simulink model "SPWM_HDLCoder_MCSI2024"  (R2021a)
settings: Solver=FixedStepDiscrete  StartTime=0.0  StopTime=0.00001  FixedStep=2.5e-8  RelTol=1e-3  EnableMultiTasking=on
undefined symbols (not defined in the file or in its folder): cfg
libraries: simulink x9, hdlsllib x8
settings Model: Creator=Damian  LastModifiedBy=Damian
settings OptimizationCC: BlockReduction=off  ConditionallyExecuteInputs=off
settings DebuggingCC: SingleTaskRateTransMsg=error

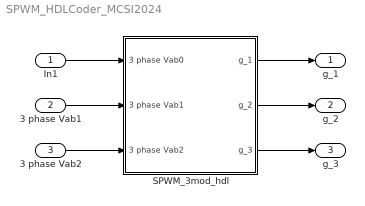
== system SPWM_HDLCoder_MCSI2024 ==
  In1 : Inport  OutDataTypeStr=fixdt(0,8,0)
  3 phase Vab1 : Inport  Port=2  OutDataTypeStr=fixdt(0,8,0)
  3 phase Vab2 : Inport  Port=3  OutDataTypeStr=fixdt(0,8,0)
  SPWM_3mod_hdl : Subsystem
  g_1 : Outport
  g_2 : Outport  Port=2
  g_3 : Outport  Port=3
  wires:
  In1/1 -> SPWM_3mod_hdl/1(3 phase Vab0)
  3 phase Vab1/1 -> SPWM_3mod_hdl/2(3 phase Vab1)
  3 phase Vab2/1 -> SPWM_3mod_hdl/3(3 phase Vab2)
  SPWM_3mod_hdl/1(g_1) -> g_1/1
  SPWM_3mod_hdl/2(g_2) -> g_2/1
  SPWM_3mod_hdl/3(g_3) -> g_3/1

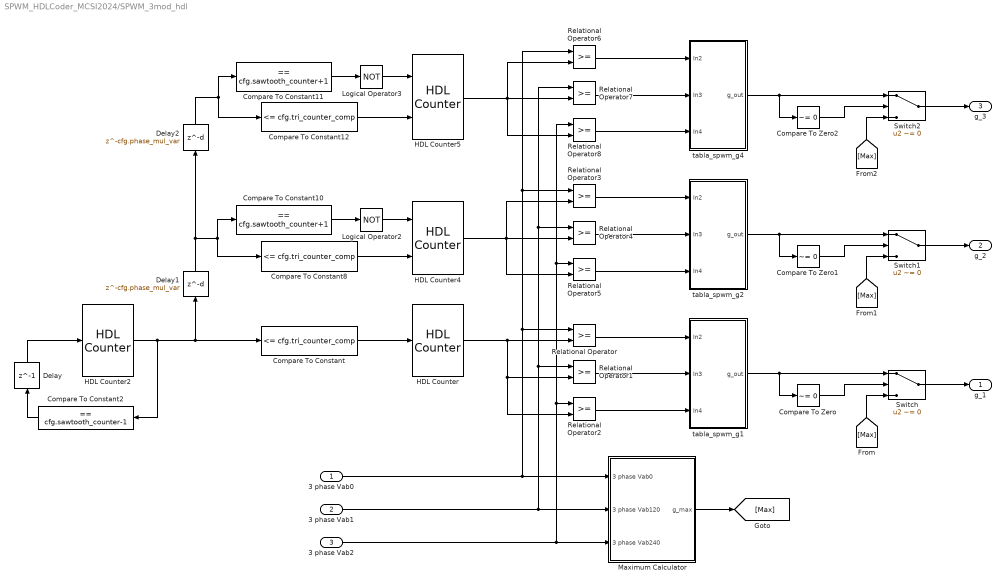
== system SPWM_HDLCoder_MCSI2024/SPWM_3mod_hdl ==
  3 phase Vab0 : Inport  OutDataTypeStr=fixdt(0,8,0)
  3 phase Vab1 : Inport  Port=2  OutDataTypeStr=fixdt(0,8,0)
  3 phase Vab2 : Inport  Port=3  OutDataTypeStr=fixdt(0,8,0)
  Compare To Constant : simulink/Logic and Bit Operations/Compare To Constant  relop=<=  const=cfg.tri_counter_comp  OutDataTypeStr=boolean
  Compare To Constant10 : simulink/Logic and Bit Operations/Compare To Constant  relop===  const=cfg.sawtooth_counter+1  OutDataTypeStr=boolean
  Compare To Constant11 : simulink/Logic and Bit Operations/Compare To Constant  relop===  const=cfg.sawtooth_counter+1  OutDataTypeStr=boolean
  Compare To Constant12 : simulink/Logic and Bit Operations/Compare To Constant  relop=<=  const=cfg.tri_counter_comp  OutDataTypeStr=boolean
  Compare To Constant2 : simulink/Logic and Bit Operations/Compare To Constant  relop===  const=cfg.sawtooth_counter-1  OutDataTypeStr=boolean
  Compare To Constant8 : simulink/Logic and Bit Operations/Compare To Constant  relop=<=  const=cfg.tri_counter_comp  OutDataTypeStr=boolean
  Compare To Zero : simulink/Logic and Bit Operations/Compare To Zero  relop=~=  OutDataTypeStr=boolean
  Compare To Zero1 : simulink/Logic and Bit Operations/Compare To Zero  relop=~=  OutDataTypeStr=boolean
  Compare To Zero2 : simulink/Logic and Bit Operations/Compare To Zero  relop=~=  OutDataTypeStr=boolean
  Delay : Delay  DelayLength=1  InitialCondition=0
  Delay1 : Delay  DelayLength=cfg.phase_mul_var  InitialCondition=cfg.sawtooth_counter+1
  Delay2 : Delay  DelayLength=cfg.phase_mul_var  InitialCondition=cfg.sawtooth_counter+1
  HDL Counter : hdlsllib/Sources/HDL Counter  CountType=Free running  CountInit=0  CountStep=1  CountMax=255  CountFromType=Initial value  CountFrom=0  CountResetPort=off  CountLoadPort=off  CountEnbPort=off  CountDirPort=on  CountHitOutputPort=off  CountDataType=Unsigned  CountWordLen=8  CountFracLen=0  CountSampTime=1
  HDL Counter2 : hdlsllib/Sources/HDL Counter  CountType=Free running  CountInit=0  CountStep=1  CountMax=cfg.sawtooth_counter-1  CountFromType=Initial value  CountFrom=0  CountResetPort=on  CountLoadPort=off  CountEnbPort=off  CountDirPort=off  CountHitOutputPort=off  CountDataType=Unsigned  CountWordLen=16  CountFracLen=0  CountSampTime=1
  HDL Counter4 : hdlsllib/Sources/HDL Counter  CountType=Free running  CountInit=0  CountStep=1  CountMax=255  CountFromType=Initial value  CountFrom=0  CountResetPort=off  CountLoadPort=off  CountEnbPort=on  CountDirPort=on  CountHitOutputPort=off  CountDataType=Unsigned  CountWordLen=8  CountFracLen=0  CountSampTime=1
  HDL Counter5 : hdlsllib/Sources/HDL Counter  CountType=Free running  CountInit=0  CountStep=1  CountMax=255  CountFromType=Initial value  CountFrom=0  CountResetPort=off  CountLoadPort=off  CountEnbPort=on  CountDirPort=on  CountHitOutputPort=off  CountDataType=Unsigned  CountWordLen=8  CountFracLen=0  CountSampTime=1
  Logical Operator2 : Logic  Operator=NOT  AllPortsSameDT=off  OutDataTypeStr=boolean
  Logical Operator3 : Logic  Operator=NOT  AllPortsSameDT=off  OutDataTypeStr=boolean
  Maximum Calculator : Subsystem
  Relational Operator{,1..8} (9 alike) : RelationalOperator  OutDataTypeStr=boolean  RndMeth=Nearest
  Switch : Switch  Criteria=u2 ~= 0
  Switch1 : Switch  Criteria=u2 ~= 0
  Switch2 : Switch  Criteria=u2 ~= 0
  tabla_spwm_g1 : Subsystem
  tabla_spwm_g2 : Subsystem
  tabla_spwm_g4 : Subsystem
  g_1 : Outport
  g_2 : Outport  Port=2
  g_3 : Outport  Port=3
  wires:
  HDL Counter4/1 -> Relational Operator4/2, Relational Operator3/2, Relational Operator5/2
  Compare To Constant12/1 -> HDL Counter5/2
  tabla_spwm_g4/1(g_out) -> Compare To Zero2/1, Switch2/1
  3 phase Vab2/1 -> Relational Operator5/1, Relational Operator8/1, Relational Operator2/1, Maximum Calculator/3(3 phase Vab240)
  Delay1/1 -> Delay2/1, Compare To Constant10/1, Compare To Constant8/1
  [Max] -> Switch/3
  Relational Operator1/1 -> tabla_spwm_g1/2(In3)
  Delay2/1 -> Compare To Constant11/1, Compare To Constant12/1
  tabla_spwm_g1/1(g_out) -> Compare To Zero/1, Switch/1
  Relational Operator/1 -> tabla_spwm_g1/1(In2)
  Relational Operator7/1 -> tabla_spwm_g4/2(In3)
  Logical Operator2/1 -> HDL Counter4/1
  Relational Operator8/1 -> tabla_spwm_g4/3(In4)
  Delay/1 -> HDL Counter2/1
  3 phase Vab1/1 -> Maximum Calculator/2(3 phase Vab120), Relational Operator1/1, Relational Operator4/1, Relational Operator7/1
  Compare To Zero2/1 -> Switch2/2
  3 phase Vab0/1 -> Maximum Calculator/1(3 phase Vab0), Relational Operator/1, Relational Operator3/1, Relational Operator6/1
  Compare To Constant2/1 -> Delay/1
  [Max] -> Switch2/3
  Switch2/1 -> g_3/1
  Maximum Calculator/1(g_max) -> [Max]
  Relational Operator6/1 -> tabla_spwm_g4/1(In2)
  HDL Counter2/1 -> Compare To Constant2/1, Delay1/1, Compare To Constant/1
  HDL Counter5/1 -> Relational Operator7/2, Relational Operator6/2, Relational Operator8/2
  HDL Counter/1 -> Relational Operator2/2, Relational Operator1/2, Relational Operator/2
  Switch/1 -> g_1/1
  Compare To Constant10/1 -> Logical Operator2/1
  Compare To Zero/1 -> Switch/2
  Relational Operator5/1 -> tabla_spwm_g2/3(In4)
  Relational Operator2/1 -> tabla_spwm_g1/3(In4)
  Compare To Constant/1 -> HDL Counter/1
  tabla_spwm_g2/1(g_out) -> Compare To Zero1/1, Switch1/1
  [Max] -> Switch1/3
  Compare To Constant8/1 -> HDL Counter4/2
  Compare To Constant11/1 -> Logical Operator3/1
  Compare To Zero1/1 -> Switch1/2
  Logical Operator3/1 -> HDL Counter5/1
  Switch1/1 -> g_2/1
  Relational Operator3/1 -> tabla_spwm_g2/1(In2)
  Relational Operator4/1 -> tabla_spwm_g2/2(In3)

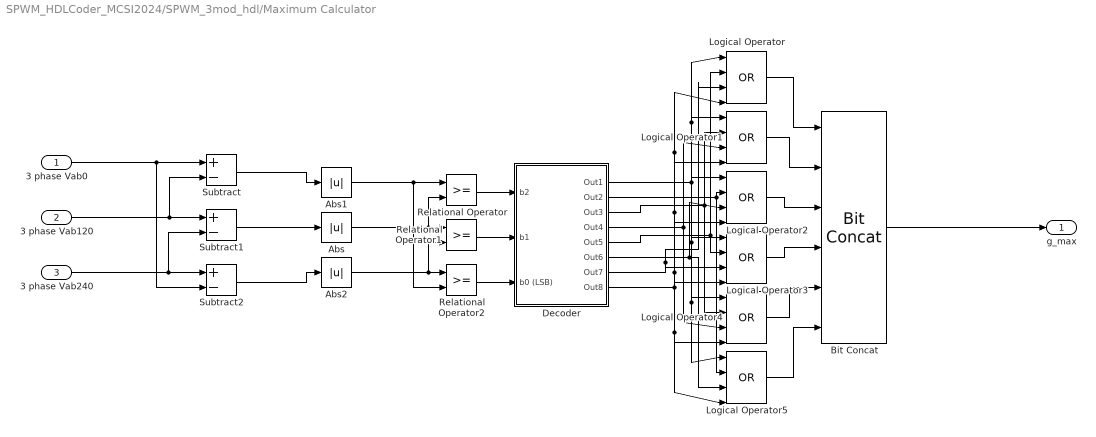
== system SPWM_HDLCoder_MCSI2024/SPWM_3mod_hdl/Maximum Calculator ==
  3 phase Vab0 : Inport
  3 phase Vab120 : Inport  Port=2
  3 phase Vab240 : Inport  Port=3
  Abs : Abs
  Abs1 : Abs
  Abs2 : Abs
  Bit Concat : hdlsllib/Logic and Bit Operations/Bit Concat  numInputs=6
  Decoder : Subsystem
  Logical Operator{,1..5} (6 alike) : Logic  Operator=OR  Inputs=4  IconShape=distinctive  AllPortsSameDT=off  OutDataTypeStr=boolean
  Relational Operator : RelationalOperator  OutDataTypeStr=boolean  RndMeth=Nearest
  Relational Operator1 : RelationalOperator  OutDataTypeStr=boolean  RndMeth=Nearest
  Relational Operator2 : RelationalOperator  OutDataTypeStr=boolean  RndMeth=Nearest
  Subtract : Sum  Inputs=+-  OutDataTypeStr=int16
  Subtract1 : Sum  Inputs=+-  OutDataTypeStr=int16
  Subtract2 : Sum  Inputs=+-  OutDataTypeStr=int16
  g_max : Outport  VectorParamsAs1DForOutWhenUnconnected=off
  wires:
  Relational Operator/1 -> Decoder/1(b2)
  Abs1/1 -> Relational Operator/1, Relational Operator2/2
  Logical Operator2/1 -> Bit Concat/3
  Abs/1 -> Relational Operator/2, Relational Operator1/1
  3 phase Vab0/1 -> Subtract2/2, Subtract/1
  Decoder/6(Out6) -> Logical Operator5/3, Logical Operator2/3
  Decoder/3(Out3) -> Logical Operator4/2, Logical Operator1/2
  Decoder/2(Out2) -> Logical Operator2/2, Logical Operator5/2
  3 phase Vab240/1 -> Subtract2/1, Subtract1/2
  Logical Operator5/1 -> Bit Concat/6
  Decoder/1(Out1) -> Logical Operator1/1, Logical Operator/1, Logical Operator5/1, Logical Operator4/1, Logical Operator3/1, Logical Operator2/1
  Abs2/1 -> Relational Operator1/2, Relational Operator2/1
  Subtract1/1 -> Abs/1
  Decoder/4(Out4) -> Logical Operator4/3, Logical Operator1/3
  3 phase Vab120/1 -> Subtract1/1, Subtract/2
  Logical Operator3/1 -> Bit Concat/4
  Decoder/5(Out5) -> Logical Operator3/2, Logical Operator/2
  Subtract/1 -> Abs1/1
  Subtract2/1 -> Abs2/1
  Relational Operator1/1 -> Decoder/2(b1)
  Relational Operator2/1 -> Decoder/3(b0 (LSB))
  Logical Operator1/1 -> Bit Concat/2
  Decoder/8(Out8) -> Logical Operator/4, Logical Operator1/4, Logical Operator2/4, Logical Operator3/4, Logical Operator4/4, Logical Operator5/4
  Decoder/7(Out7) -> Logical Operator3/3, Logical Operator/3
  Logical Operator4/1 -> Bit Concat/5
  Logical Operator/1 -> Bit Concat/1
  Bit Concat/1 -> g_max/1

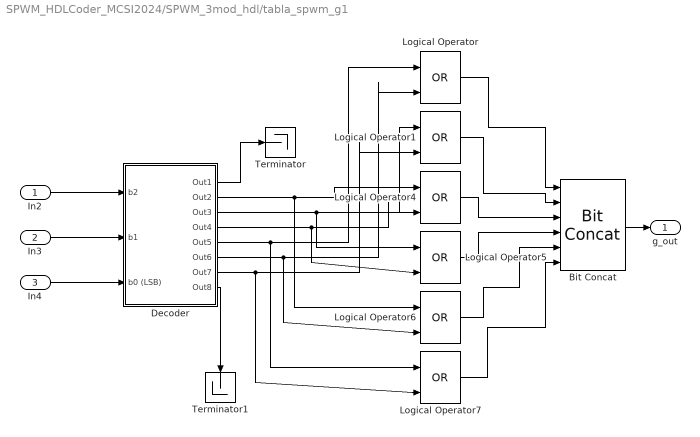
== system SPWM_HDLCoder_MCSI2024/SPWM_3mod_hdl/tabla_spwm_g1 ==
  In2 : Inport
  In3 : Inport  Port=2
  In4 : Inport  Port=3
  Bit Concat : hdlsllib/Logic and Bit Operations/Bit Concat  numInputs=6
  Decoder : Subsystem
  Logical Operator{,1,4..7} (6 alike) : Logic  Operator=OR  IconShape=distinctive  AllPortsSameDT=off  OutDataTypeStr=boolean
  Terminator : Terminator
  Terminator1 : Terminator
  g_out : Outport  VectorParamsAs1DForOutWhenUnconnected=off
  wires:
  Decoder/7(Out7) -> Logical Operator1/2, Logical Operator7/2
  Logical Operator4/1 -> Bit Concat/3
  Logical Operator/1 -> Bit Concat/1
  Logical Operator1/1 -> Bit Concat/2
  Decoder/2(Out2) -> Logical Operator4/1, Logical Operator6/1
  Logical Operator7/1 -> Bit Concat/6
  Logical Operator5/1 -> Bit Concat/4
  Decoder/5(Out5) -> Logical Operator/1, Logical Operator7/1
  Logical Operator6/1 -> Bit Concat/5
  In4/1 -> Decoder/3(b0 (LSB))
  In3/1 -> Decoder/2(b1)
  In2/1 -> Decoder/1(b2)
  Decoder/4(Out4) -> Logical Operator5/2, Logical Operator4/2
  Decoder/3(Out3) -> Logical Operator5/1, Logical Operator1/1
  Decoder/6(Out6) -> Logical Operator/2, Logical Operator6/2
  Decoder/1(Out1) -> Terminator/1
  Decoder/8(Out8) -> Terminator1/1
  Bit Concat/1 -> g_out/1

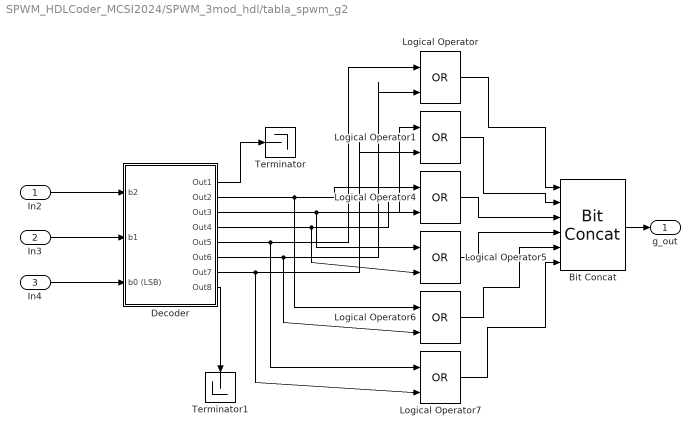
== system SPWM_HDLCoder_MCSI2024/SPWM_3mod_hdl/tabla_spwm_g2 ==
  In2 : Inport
  In3 : Inport  Port=2
  In4 : Inport  Port=3
  Bit Concat : hdlsllib/Logic and Bit Operations/Bit Concat  numInputs=6
  Decoder : Subsystem
  Logical Operator{,1,4..7} (6 alike) : Logic  Operator=OR  IconShape=distinctive  AllPortsSameDT=off  OutDataTypeStr=boolean
  Terminator : Terminator
  Terminator1 : Terminator
  g_out : Outport  VectorParamsAs1DForOutWhenUnconnected=off
  wires:
  Decoder/7(Out7) -> Logical Operator1/2, Logical Operator7/2
  Logical Operator4/1 -> Bit Concat/3
  Logical Operator/1 -> Bit Concat/1
  Logical Operator1/1 -> Bit Concat/2
  Decoder/2(Out2) -> Logical Operator4/1, Logical Operator6/1
  Logical Operator7/1 -> Bit Concat/6
  Logical Operator5/1 -> Bit Concat/4
  Decoder/5(Out5) -> Logical Operator/1, Logical Operator7/1
  Logical Operator6/1 -> Bit Concat/5
  In4/1 -> Decoder/3(b0 (LSB))
  In3/1 -> Decoder/2(b1)
  In2/1 -> Decoder/1(b2)
  Decoder/4(Out4) -> Logical Operator5/2, Logical Operator4/2
  Decoder/3(Out3) -> Logical Operator5/1, Logical Operator1/1
  Decoder/6(Out6) -> Logical Operator/2, Logical Operator6/2
  Decoder/1(Out1) -> Terminator/1
  Decoder/8(Out8) -> Terminator1/1
  Bit Concat/1 -> g_out/1

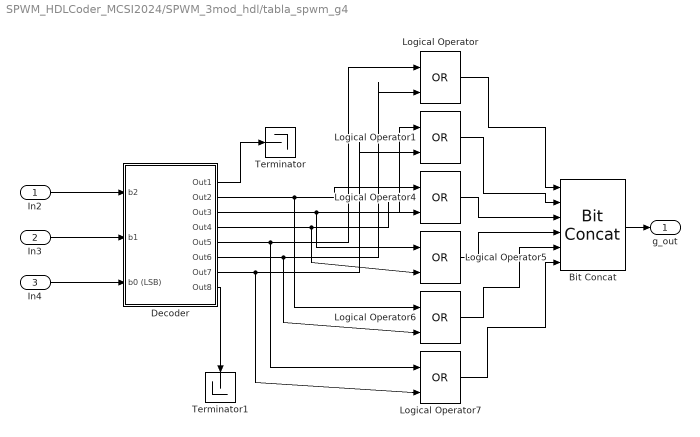
== system SPWM_HDLCoder_MCSI2024/SPWM_3mod_hdl/tabla_spwm_g4 ==
  In2 : Inport
  In3 : Inport  Port=2
  In4 : Inport  Port=3
  Bit Concat : hdlsllib/Logic and Bit Operations/Bit Concat  numInputs=6
  Decoder : Subsystem
  Logical Operator{,1,4..7} (6 alike) : Logic  Operator=OR  IconShape=distinctive  AllPortsSameDT=off  OutDataTypeStr=boolean
  Terminator : Terminator
  Terminator1 : Terminator
  g_out : Outport  VectorParamsAs1DForOutWhenUnconnected=off
  wires:
  Decoder/7(Out7) -> Logical Operator1/2, Logical Operator7/2
  Logical Operator4/1 -> Bit Concat/3
  Logical Operator/1 -> Bit Concat/1
  Logical Operator1/1 -> Bit Concat/2
  Decoder/2(Out2) -> Logical Operator4/1, Logical Operator6/1
  Logical Operator7/1 -> Bit Concat/6
  Logical Operator5/1 -> Bit Concat/4
  Decoder/5(Out5) -> Logical Operator/1, Logical Operator7/1
  Logical Operator6/1 -> Bit Concat/5
  In4/1 -> Decoder/3(b0 (LSB))
  In3/1 -> Decoder/2(b1)
  In2/1 -> Decoder/1(b2)
  Decoder/4(Out4) -> Logical Operator5/2, Logical Operator4/2
  Decoder/3(Out3) -> Logical Operator5/1, Logical Operator1/1
  Decoder/6(Out6) -> Logical Operator/2, Logical Operator6/2
  Decoder/1(Out1) -> Terminator/1
  Decoder/8(Out8) -> Terminator1/1
  Bit Concat/1 -> g_out/1

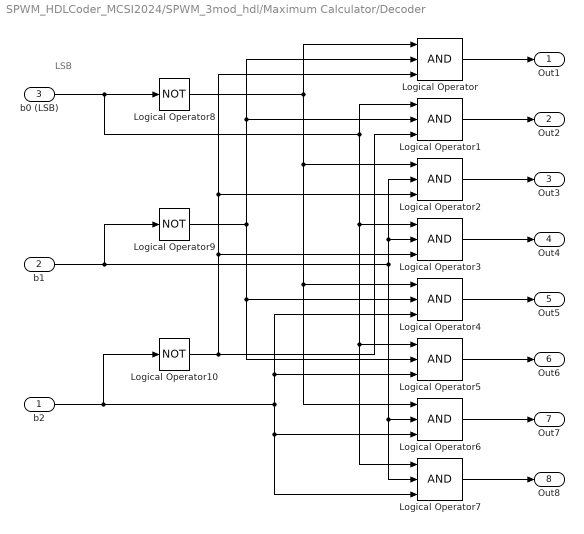
== system SPWM_HDLCoder_MCSI2024/SPWM_3mod_hdl/Maximum Calculator/Decoder ==
  note: LSB
  b2 : Inport
  b1 : Inport  Port=2
  b0 (LSB) : Inport  Port=3
  Logical Operator{,1..7} (8 alike) : Logic  Inputs=3  IconShape=distinctive  AllPortsSameDT=off  OutDataTypeStr=boolean
  Logical Operator10 : Logic  Operator=NOT  IconShape=distinctive  AllPortsSameDT=off  OutDataTypeStr=boolean
  Logical Operator8 : Logic  Operator=NOT  IconShape=distinctive  AllPortsSameDT=off  OutDataTypeStr=boolean
  Logical Operator9 : Logic  Operator=NOT  IconShape=distinctive  AllPortsSameDT=off  OutDataTypeStr=boolean
  Out1 : Outport
  Out2 : Outport  Port=2
  Out3 : Outport  Port=3
  Out4 : Outport  Port=4
  Out5 : Outport  Port=5
  Out6 : Outport  Port=6
  Out7 : Outport  Port=7
  Out8 : Outport  Port=8
  wires:
  Logical Operator9/1 -> Logical Operator5/2, Logical Operator4/2, Logical Operator1/2, Logical Operator/2
  Logical Operator5/1 -> Out6/1
  Logical Operator1/1 -> Out2/1
  Logical Operator10/1 -> Logical Operator3/3, Logical Operator2/3, Logical Operator/3, Logical Operator1/3
  Logical Operator/1 -> Out1/1
  Logical Operator8/1 -> Logical Operator6/1, Logical Operator4/1, Logical Operator2/1, Logical Operator/1
  b2/1 -> Logical Operator4/3, Logical Operator5/3, Logical Operator7/3, Logical Operator6/3, Logical Operator10/1
  b0 (LSB)/1 -> Logical Operator7/1, Logical Operator5/1, Logical Operator3/1, Logical Operator1/1, Logical Operator8/1
  Logical Operator7/1 -> Out8/1
  b1/1 -> Logical Operator3/2, Logical Operator2/2, Logical Operator7/2, Logical Operator6/2, Logical Operator9/1
  Logical Operator4/1 -> Out5/1
  Logical Operator6/1 -> Out7/1
  Logical Operator3/1 -> Out4/1
  Logical Operator2/1 -> Out3/1

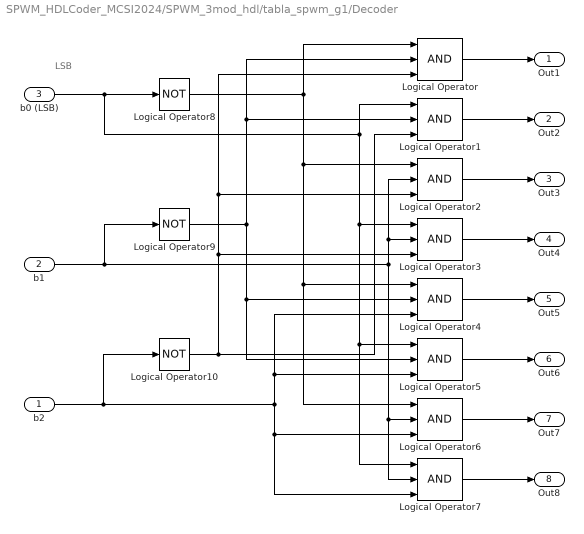
== system SPWM_HDLCoder_MCSI2024/SPWM_3mod_hdl/tabla_spwm_g1/Decoder ==
  note: LSB
  b2 : Inport
  b1 : Inport  Port=2
  b0 (LSB) : Inport  Port=3
  Logical Operator{,1..7} (8 alike) : Logic  Inputs=3  IconShape=distinctive  AllPortsSameDT=off  OutDataTypeStr=boolean
  Logical Operator10 : Logic  Operator=NOT  IconShape=distinctive  AllPortsSameDT=off  OutDataTypeStr=boolean
  Logical Operator8 : Logic  Operator=NOT  IconShape=distinctive  AllPortsSameDT=off  OutDataTypeStr=boolean
  Logical Operator9 : Logic  Operator=NOT  IconShape=distinctive  AllPortsSameDT=off  OutDataTypeStr=boolean
  Out1 : Outport
  Out2 : Outport  Port=2
  Out3 : Outport  Port=3
  Out4 : Outport  Port=4
  Out5 : Outport  Port=5
  Out6 : Outport  Port=6
  Out7 : Outport  Port=7
  Out8 : Outport  Port=8
  wires:
  Logical Operator9/1 -> Logical Operator5/2, Logical Operator4/2, Logical Operator1/2, Logical Operator/2
  Logical Operator5/1 -> Out6/1
  Logical Operator1/1 -> Out2/1
  Logical Operator10/1 -> Logical Operator3/3, Logical Operator2/3, Logical Operator/3, Logical Operator1/3
  Logical Operator/1 -> Out1/1
  Logical Operator8/1 -> Logical Operator6/1, Logical Operator4/1, Logical Operator2/1, Logical Operator/1
  b2/1 -> Logical Operator4/3, Logical Operator5/3, Logical Operator7/3, Logical Operator6/3, Logical Operator10/1
  b0 (LSB)/1 -> Logical Operator7/1, Logical Operator5/1, Logical Operator3/1, Logical Operator1/1, Logical Operator8/1
  Logical Operator7/1 -> Out8/1
  b1/1 -> Logical Operator3/2, Logical Operator2/2, Logical Operator7/2, Logical Operator6/2, Logical Operator9/1
  Logical Operator4/1 -> Out5/1
  Logical Operator6/1 -> Out7/1
  Logical Operator3/1 -> Out4/1
  Logical Operator2/1 -> Out3/1

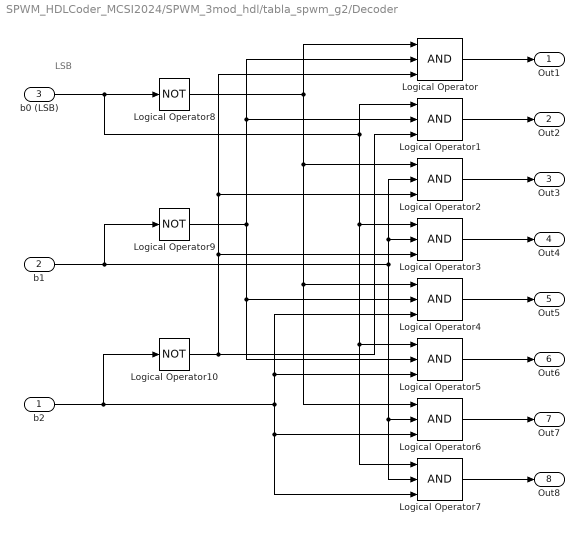
== system SPWM_HDLCoder_MCSI2024/SPWM_3mod_hdl/tabla_spwm_g2/Decoder ==
  note: LSB
  b2 : Inport
  b1 : Inport  Port=2
  b0 (LSB) : Inport  Port=3
  Logical Operator{,1..7} (8 alike) : Logic  Inputs=3  IconShape=distinctive  AllPortsSameDT=off  OutDataTypeStr=boolean
  Logical Operator10 : Logic  Operator=NOT  IconShape=distinctive  AllPortsSameDT=off  OutDataTypeStr=boolean
  Logical Operator8 : Logic  Operator=NOT  IconShape=distinctive  AllPortsSameDT=off  OutDataTypeStr=boolean
  Logical Operator9 : Logic  Operator=NOT  IconShape=distinctive  AllPortsSameDT=off  OutDataTypeStr=boolean
  Out1 : Outport
  Out2 : Outport  Port=2
  Out3 : Outport  Port=3
  Out4 : Outport  Port=4
  Out5 : Outport  Port=5
  Out6 : Outport  Port=6
  Out7 : Outport  Port=7
  Out8 : Outport  Port=8
  wires:
  Logical Operator9/1 -> Logical Operator5/2, Logical Operator4/2, Logical Operator1/2, Logical Operator/2
  Logical Operator5/1 -> Out6/1
  Logical Operator1/1 -> Out2/1
  Logical Operator10/1 -> Logical Operator3/3, Logical Operator2/3, Logical Operator/3, Logical Operator1/3
  Logical Operator/1 -> Out1/1
  Logical Operator8/1 -> Logical Operator6/1, Logical Operator4/1, Logical Operator2/1, Logical Operator/1
  b2/1 -> Logical Operator4/3, Logical Operator5/3, Logical Operator7/3, Logical Operator6/3, Logical Operator10/1
  b0 (LSB)/1 -> Logical Operator7/1, Logical Operator5/1, Logical Operator3/1, Logical Operator1/1, Logical Operator8/1
  Logical Operator7/1 -> Out8/1
  b1/1 -> Logical Operator3/2, Logical Operator2/2, Logical Operator7/2, Logical Operator6/2, Logical Operator9/1
  Logical Operator4/1 -> Out5/1
  Logical Operator6/1 -> Out7/1
  Logical Operator3/1 -> Out4/1
  Logical Operator2/1 -> Out3/1

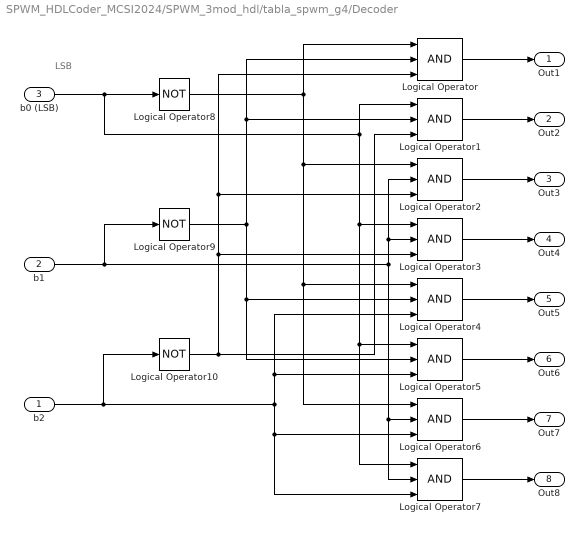
== system SPWM_HDLCoder_MCSI2024/SPWM_3mod_hdl/tabla_spwm_g4/Decoder ==
  note: LSB
  b2 : Inport
  b1 : Inport  Port=2
  b0 (LSB) : Inport  Port=3
  Logical Operator{,1..7} (8 alike) : Logic  Inputs=3  IconShape=distinctive  AllPortsSameDT=off  OutDataTypeStr=boolean
  Logical Operator10 : Logic  Operator=NOT  IconShape=distinctive  AllPortsSameDT=off  OutDataTypeStr=boolean
  Logical Operator8 : Logic  Operator=NOT  IconShape=distinctive  AllPortsSameDT=off  OutDataTypeStr=boolean
  Logical Operator9 : Logic  Operator=NOT  IconShape=distinctive  AllPortsSameDT=off  OutDataTypeStr=boolean
  Out1 : Outport
  Out2 : Outport  Port=2
  Out3 : Outport  Port=3
  Out4 : Outport  Port=4
  Out5 : Outport  Port=5
  Out6 : Outport  Port=6
  Out7 : Outport  Port=7
  Out8 : Outport  Port=8
  wires:
  Logical Operator9/1 -> Logical Operator5/2, Logical Operator4/2, Logical Operator1/2, Logical Operator/2
  Logical Operator5/1 -> Out6/1
  Logical Operator1/1 -> Out2/1
  Logical Operator10/1 -> Logical Operator3/3, Logical Operator2/3, Logical Operator/3, Logical Operator1/3
  Logical Operator/1 -> Out1/1
  Logical Operator8/1 -> Logical Operator6/1, Logical Operator4/1, Logical Operator2/1, Logical Operator/1
  b2/1 -> Logical Operator4/3, Logical Operator5/3, Logical Operator7/3, Logical Operator6/3, Logical Operator10/1
  b0 (LSB)/1 -> Logical Operator7/1, Logical Operator5/1, Logical Operator3/1, Logical Operator1/1, Logical Operator8/1
  Logical Operator7/1 -> Out8/1
  b1/1 -> Logical Operator3/2, Logical Operator2/2, Logical Operator7/2, Logical Operator6/2, Logical Operator9/1
  Logical Operator4/1 -> Out5/1
  Logical Operator6/1 -> Out7/1
  Logical Operator3/1 -> Out4/1
  Logical Operator2/1 -> Out3/1
